simulink subsystem "PX4_Control_FixedWing"  (R2025a)
settings: Solver=VariableStepAuto  StartTime=0.0  StopTime=10.0  RelTol=1e-3
libraries: px4uORBlib x2
settings Model: Creator=gurt1  LastModifiedBy=17036

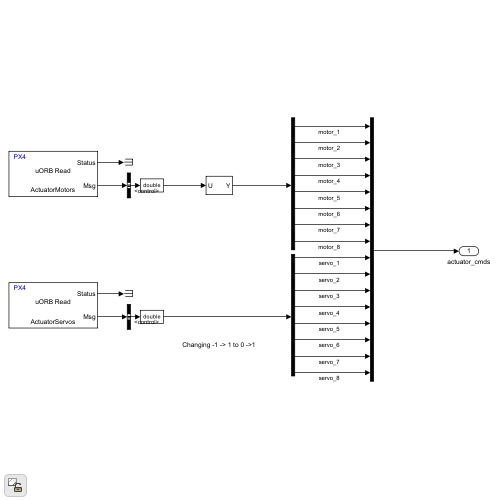
[thumbnail: Simulink's stored preview of the top-level diagram]
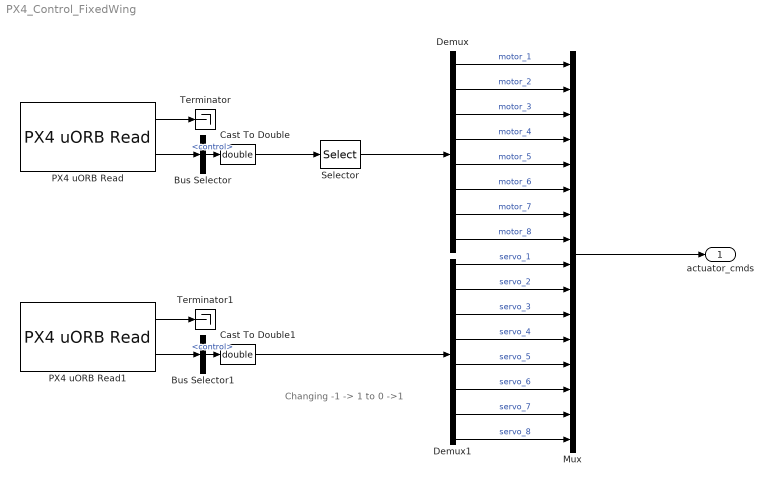
== system PX4_Control_FixedWing ==
  note: Changing -1 -> 1 to 0 ->1
  Bus Selector : BusSelector  OutputSignals=control
  Bus Selector1 : BusSelector  OutputSignals=control
  Cast To Double : DataTypeConversion  OutDataTypeStr=double  SaturateOnIntegerOverflow=off  RndMeth=Floor
  Cast To Double1 : DataTypeConversion  OutDataTypeStr=double  SaturateOnIntegerOverflow=off  RndMeth=Floor
  Demux : Demux  Outputs=8
  Demux1 : Demux  Outputs=8
  Mux : Mux  Inputs=16
  PX4 uORB Read : px4uORBlib/PX4 uORB Read  uORBTopic=ActuatorMotors  selectInstance=ActuatorMotors  SampleTime=-1  BlockingMode=off  BlockTimeout=1e-3
  PX4 uORB Read1 : px4uORBlib/PX4 uORB Read  uORBTopic=ActuatorServos  selectInstance=ActuatorServos  SampleTime=-1  BlockingMode=off  BlockTimeout=1e-3
  Selector : Selector  InputPortWidth=12  IndexOptions=Index vector (dialog)  Indices=[1:8]  OutputSizes=1
  Terminator : Terminator
  Terminator1 : Terminator
  actuator_cmds : Outport
  wires:
  Mux/1 -> actuator_cmds/1
  PX4 uORB Read/1 -> Terminator/1
  PX4 uORB Read/2 -> Bus Selector/1
  PX4 uORB Read1/1 -> Terminator1/1
  PX4 uORB Read1/2 -> Bus Selector1/1
  Bus Selector1/1 -> Cast To Double1/1  "<control>"
  Demux/1 -> Mux/1  "motor_1"
  Demux/2 -> Mux/2  "motor_2"
  Demux/3 -> Mux/3  "motor_3"
  Demux/4 -> Mux/4  "motor_4"
  Demux/5 -> Mux/5  "motor_5"
  Demux/6 -> Mux/6  "motor_6"
  Demux/7 -> Mux/7  "motor_7"
  Demux/8 -> Mux/8  "motor_8"
  Bus Selector/1 -> Cast To Double/1  "<control>"
  Demux1/1 -> Mux/9  "servo_1"
  Demux1/2 -> Mux/10  "servo_2"
  Demux1/3 -> Mux/11  "servo_3"
  Demux1/4 -> Mux/12  "servo_4"
  Demux1/5 -> Mux/13  "servo_5"
  Demux1/6 -> Mux/14  "servo_6"
  Demux1/7 -> Mux/15  "servo_7"
  Demux1/8 -> Mux/16  "servo_8"
  Cast To Double/1 -> Selector/1
  Cast To Double1/1 -> Demux1/1
  Selector/1 -> Demux/1
